simulink model "TargetSpeedThrottle"  (R2021a)
settings: Solver=FixedStepDiscrete  StartTime=0.0  StopTime=10.0  FixedStep=0.01  RelTol=1e-3
undefined symbols (not defined in the file): DiscIntNeverNeededParam, Kp, opMode, target_dec_hold, target_dec_short, target_inc_hold, target_inc_short, throt_max, throt_min, Ts, tsp_max, tsp_min
libraries: simulink x7
settings Model: RequirementInfo={} %GIDa_1a3689c1_601b_4931_a17a_efea0d5071ba  DataDictionary=crs_controllerdic.sldd  EnableAccessToBaseWorkspace=off  Creator=The MathWorks, Inc.  LastModifiedBy=shayashi
settings SolverCC: AlgebraicLoopSolver=TrustRegion
settings DataIOCC: SaveOutput=off  SignalLogging=off  DSMLogging=off  SaveTime=off  ReturnWorkspaceOutputs=off
settings OptimizationCC: DefaultParameterBehavior=Inlined  PassReuseOutputArgsAs=Individual arguments  EfficientTunableParamExpr=on
settings DebuggingCC: ParameterTunabilityLossMsg=error  SFMachineParentedDataDiag=warning  ArithmeticOperatorsInVariantConditions=warning
settings SFSimCC: SimUseLocalCustomCode=off  CustomCodeUndefinedFunction=UseInterfaceOnly
settings RTWCC: SystemTargetFile=ert.tlc  GenCodeOnly=on  TemplateMakefile=ert_default_tmf  GenerateReport=on  RTWUseLocalCustomCode=off  IncludeHyperlinkInReport=on  LaunchReport=on  GenerateTraceInfo=on  GenerateTraceReport=on  GenerateTraceReportSl=on  GenerateTraceReportSf=on  GenerateTraceReportEml=on
settings CodeAppCC: ForceParamTrailComments=on  IgnoreCustomStorageClasses=off  OperatorAnnotations=on  SimulinkDataObjDesc=on  SFDataObjDesc=on  MATLABFcnDesc=on  InsertBlockDesc=on  StateflowObjectComments=on  MATLABSourceComments=on  ReqsInCode=on
settings ERTTargetCC: TargetLangStandard=C99 (ISO)  GenerateSampleERTMain=on  InlinedParameterPlacement=NonHierarchical  ERTCustomFileTemplate=example_file_process.tlc
settings ConfigComp: DVTestSuiteOptimization=Auto  DVDetectOutOfBounds=on

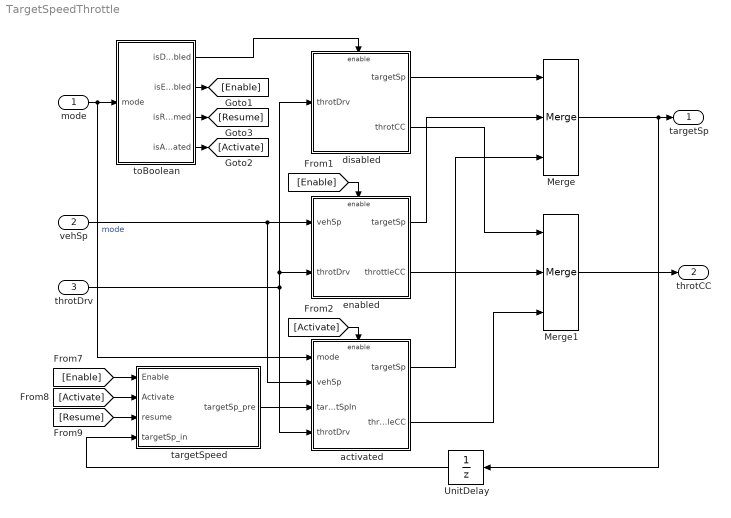
== system TargetSpeedThrottle ==
  mode : Inport  RequirementInfo={} %GIDa_22885af7_b22a_44fa_aa4d_017be81ce3db  OutDataTypeStr=Enum: opMode  PortDimensions=1  SampleTime=[0.01,0]
  vehSp : Inport  RequirementInfo={} %GIDa_f5c97d85_f23b_4cf3_86c5_8760a45faeb2  Port=2  OutDataTypeStr=double  PortDimensions=1  SampleTime=[0.01,0]
  throtDrv : Inport  RequirementInfo={} %GIDa_53068002_6435_432c_bd84_5ec1757fd185  Port=3  OutDataTypeStr=double  PortDimensions=1  SampleTime=[0.01,0]
  Merge : Merge  RequirementInfo={} %GIDa_cdca348c_f4ee_415b_942c_f6cd5980ed22  Inputs=3
  Merge1 : Merge  RequirementInfo={} %GIDa_34b46d63_1e8a_4844_895f_7afabcfedfbe  Inputs=3
  UnitDelay : UnitDelay  RequirementInfo={} %GIDa_36ca9bee_c418_49b5_b025_5c47d96671ca  SampleTime=-1  HasFrameUpgradeWarning=on
      settings: AttributesFormatString=Init = %<InitialCondition>
  activated : Subsystem  RequirementInfo={} %GIDa_d3fc8234_37e6_4215_9250_2cfb9e78a153  TreatAsAtomicUnit=on
  disabled : Subsystem  RequirementInfo={} %GIDa_06140de0_e8d8_402c_b038_77cf0712a248  TreatAsAtomicUnit=on
  enabled : Subsystem  RequirementInfo={} %GIDa_3f53baab_40ad_4365_8baf_4957a2682033  TreatAsAtomicUnit=on
  targetSpeed : Subsystem  RequirementInfo={} %GIDa_cb3d74aa_bbef_46cf_9d83_92915d058f40
  toBoolean : Subsystem  RequirementInfo={} %GIDa_708419c1_1127_4954_9632_16e4105ce24a
  targetSp : Outport  RequirementInfo={} %GIDa_29007791_7843_4644_8d92_505ff71faba5  OutDataTypeStr=double  PortDimensions=1  SampleTime=[0.01,0]  VectorParamsAs1DForOutWhenUnconnected=off
  throtCC : Outport  RequirementInfo={} %GIDa_070a8361_0cd1_420b_a715_f329e916e1ad  Port=2  OutDataTypeStr=double  PortDimensions=1  SampleTime=[0.01,0]  VectorParamsAs1DForOutWhenUnconnected=off
  wires:
  [Activate] -> targetSpeed/2(Activate)
  [Enable] -> targetSpeed/1(Enable)
  targetSpeed/1(targetSp_pre) -> activated/3(targetSpIn)
  mode/1 -> activated/1(mode), toBoolean/1(mode)  "mode"
  [Activate] -> activated/Enable
  [Enable] -> enabled/Enable
  toBoolean/1(isDisabled) -> disabled/Enable
  UnitDelay/1 -> targetSpeed/4(targetSp_in)
  Merge/1 -> UnitDelay/1, targetSp/1
  throtDrv/1 -> activated/4(throtDrv), enabled/2(throtDrv), disabled/1(throtDrv)
  vehSp/1 -> enabled/1(vehSp), activated/2(vehSp)
  toBoolean/2(isEnabled) -> [Enable]
  toBoolean/3(isResumed) -> [Resume]
  toBoolean/4(isActivated) -> [Activate]
  [Resume] -> targetSpeed/3(resume)
  disabled/1(targetSp) -> Merge/1
  enabled/1(targetSp) -> Merge/2
  activated/1(targetSp) -> Merge/3
  activated/2(throttleCC) -> Merge1/3
  enabled/2(throttleCC) -> Merge1/2
  disabled/2(throtCC) -> Merge1/1
  Merge1/1 -> throtCC/1

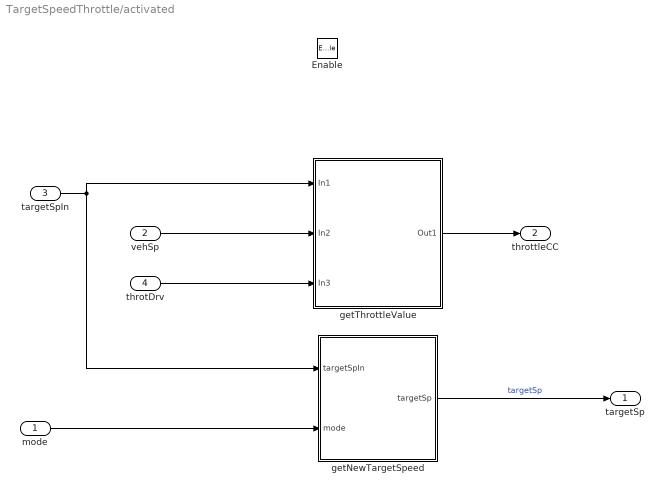
== system TargetSpeedThrottle/activated ==
  mode : Inport  RequirementInfo={} %GIDa_64384464_a4fb_41bc_9e66_5cfe7553856c
  vehSp : Inport  RequirementInfo={} %GIDa_54e68108_b78c_4afe_bc67_449efdb277bd  Port=2
  targetSpIn : Inport  RequirementInfo={} %GIDa_feedb564_4ae2_4bad_9ab3_cf1210728889  Port=3
  throtDrv : Inport  RequirementInfo={} %GIDa_834fa2e2_d354_4482_989f_6165ef52fb64  Port=4
  Enable : EnablePort  RequirementInfo={} %GIDa_bd587e7b_2324_4a3e_a90d_e93b85140e69
  getNewTargetSpeed : Subsystem  RequirementInfo={} %GIDa_cb2db30c_40f4_4c69_83f3_f6a6c8c4dbbc
  getThrottleValue : Subsystem  RequirementInfo={} %GIDa_30fb74e3_5bea_4a48_8902_fa86193af843
  targetSp : Outport  RequirementInfo={} %GIDa_4f1af6e7_9967_48df_a5c8_7598c889d755  VectorParamsAs1DForOutWhenUnconnected=off
  throttleCC : Outport  RequirementInfo={} %GIDa_61cc87ec_8da1_409c_a066_e137f06790c0  Port=2  VectorParamsAs1DForOutWhenUnconnected=off
  wires:
  getThrottleValue/1(Out1) -> throttleCC/1
  throtDrv/1 -> getThrottleValue/3(In3)
  vehSp/1 -> getThrottleValue/2(In2)
  getNewTargetSpeed/1(targetSp) -> targetSp/1  "targetSp"
  mode/1 -> getNewTargetSpeed/2(mode)
  targetSpIn/1 -> getNewTargetSpeed/1(targetSpIn), getThrottleValue/1(In1)

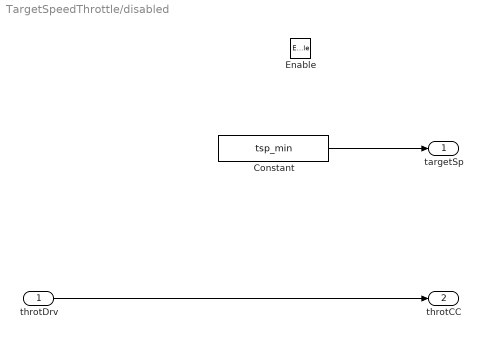
== system TargetSpeedThrottle/disabled ==
  throtDrv : Inport  RequirementInfo={} %GIDa_6cc9cf71_2141_4b22_a535_628638b2431f
  Enable : EnablePort  RequirementInfo={} %GIDa_12e821c3_8a9d_4a2d_ae26_f8ea4cd80d03
  Constant : Constant  RequirementInfo={} %GIDa_549ea7b0_4d18_4b4b_b86d_6f4ed7933c4d  Value=tsp_min  OutDataTypeStr=Inherit: Inherit via back propagation
  targetSp : Outport  RequirementInfo={} %GIDa_cfb9ce1a_28c4_4b9c_a057_b42ee2940ceb  VectorParamsAs1DForOutWhenUnconnected=off
  throtCC : Outport  RequirementInfo={} %GIDa_b0b7c855_10e5_48f0_a23b_03d9ab7ebd64  Port=2  VectorParamsAs1DForOutWhenUnconnected=off
  wires:
  throtDrv/1 -> throtCC/1
  Constant/1 -> targetSp/1

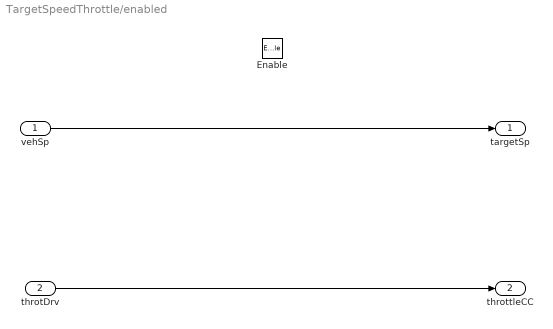
== system TargetSpeedThrottle/enabled ==
  vehSp : Inport  RequirementInfo={} %GIDa_051cacd1_d8f3_45f0_98cd_ed6e0d7dd9aa
  throtDrv : Inport  RequirementInfo={} %GIDa_4482214a_b082_4025_affc_42904b284b10  Port=2
  Enable : EnablePort  RequirementInfo={} %GIDa_6682126c_96c9_4657_ae5d_14402d8b3ec1
  targetSp : Outport  RequirementInfo={} %GIDa_6209277a_e70a_46cf_9111_d4ad6ceba119  VectorParamsAs1DForOutWhenUnconnected=off
  throttleCC : Outport  RequirementInfo={} %GIDa_5cd745c9_300b_4598_b460_5fe843c280e4  Port=2  VectorParamsAs1DForOutWhenUnconnected=off
  wires:
  throtDrv/1 -> throttleCC/1
  vehSp/1 -> targetSp/1

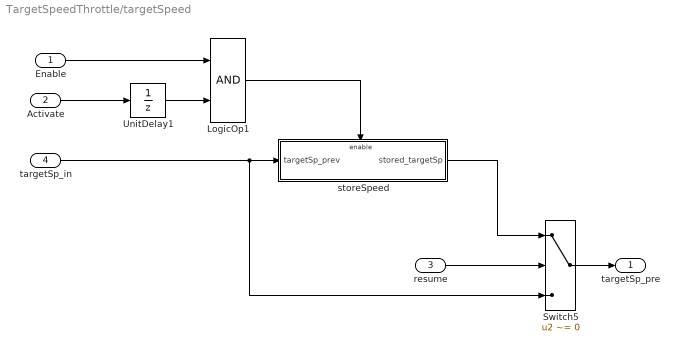
== system TargetSpeedThrottle/targetSpeed ==
  Enable : Inport  RequirementInfo={} %GIDa_fce2bafd_f2de_42bd_8112_e657c8fe1477
  Activate : Inport  RequirementInfo={} %GIDa_8a860952_06c5_4d89_b310_dabeeaa78df6  Port=2
  resume : Inport  RequirementInfo={} %GIDa_d24781cb_7428_4781_b55e_e26f6e81c793  Port=3
  targetSp_in : Inport  RequirementInfo={} %GIDa_97c5bf71_ad17_419d_a89a_c68daaf71e8b  Port=4
  LogicOp1 : Logic  RequirementInfo={} %GIDa_9c82f171_f4c6_4d19_9b0e_13b686137bc8  AllPortsSameDT=off  OutDataTypeStr=boolean
  Switch5 : Switch  RequirementInfo={} %GIDa_9efa5802_f260_41d2_9ca5_821b46ab96a6  Criteria=u2 ~= 0
  UnitDelay1 : UnitDelay  RequirementInfo={} %GIDa_adabed4e_2068_480c_8557_03c012030ff1  InitialCondition=false  SampleTime=-1  HasFrameUpgradeWarning=on
      settings: AttributesFormatString=Init = %<InitialCondition>
  storeSpeed : Subsystem  RequirementInfo={} %GIDa_21626e59_d900_4aed_83eb_aaced630845b  TreatAsAtomicUnit=on
  targetSp_pre : Outport  RequirementInfo={} %GIDa_7bb45878_dbc3_4fb7_871d_d80e6eee27c9  VectorParamsAs1DForOutWhenUnconnected=off
  wires:
  Switch5/1 -> targetSp_pre/1
  targetSp_in/1 -> storeSpeed/1(targetSp_prev), Switch5/3
  resume/1 -> Switch5/2
  Enable/1 -> LogicOp1/1
  LogicOp1/1 -> storeSpeed/Enable
  UnitDelay1/1 -> LogicOp1/2
  Activate/1 -> UnitDelay1/1
  storeSpeed/1(stored_targetSp) -> Switch5/1

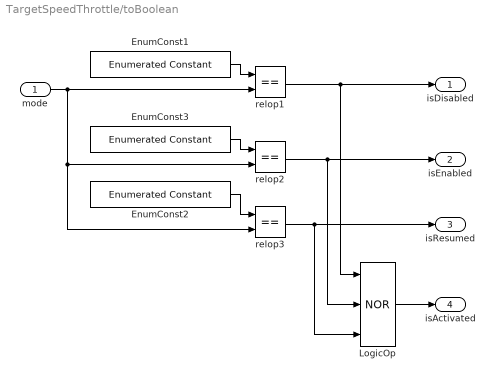
== system TargetSpeedThrottle/toBoolean ==
  mode : Inport  RequirementInfo={} %GIDa_e7e444c0_3529_4ed5_81ce_f617e2024f02
  EnumConst1 : simulink/Sources/Enumerated Constant  RequirementInfo={} %GIDa_27a9e84b_6b36_4c12_aa93_aca0a05eed93  OutDataTypeStr=Enum: opMode  Value=opMode.Disable  SampleTime=inf
  EnumConst2 : simulink/Sources/Enumerated Constant  RequirementInfo={} %GIDa_d37b8a40_9443_4f54_8bef_716a0ad75842  OutDataTypeStr=Enum: opMode  Value=opMode.Resume  SampleTime=inf
  EnumConst3 : simulink/Sources/Enumerated Constant  RequirementInfo={} %GIDa_e76c0d8e_43de_4bf9_b183_6cfd99518f27  OutDataTypeStr=Enum: opMode  Value=opMode.Enable  SampleTime=inf
  LogicOp : Logic  RequirementInfo={} %GIDa_c0c1558f_e301_4739_9f83_d240660de869  Operator=NOR  Inputs=3  AllPortsSameDT=off  OutDataTypeStr=boolean
  relop1 : RelationalOperator  RequirementInfo={} %GIDa_8114262e_aab4_4130_b326_8c0e06239675  Operator===  OutDataTypeStr=boolean  RndMeth=Nearest
  relop2 : RelationalOperator  RequirementInfo={} %GIDa_f220986f_8ed3_4e7b_a738_7af982ee01f8  Operator===  OutDataTypeStr=boolean  RndMeth=Nearest
  relop3 : RelationalOperator  RequirementInfo={} %GIDa_2bb1450f_1cf8_4106_805d_3854b6e18c7a  Operator===  OutDataTypeStr=boolean  RndMeth=Nearest
  isDisabled : Outport  RequirementInfo={} %GIDa_0a060732_89ab_4bb9_8b58_ea59ba79c186  VectorParamsAs1DForOutWhenUnconnected=off
  isEnabled : Outport  RequirementInfo={} %GIDa_daac9f50_969b_4fdf_9786_3d46f846d53d  Port=2  VectorParamsAs1DForOutWhenUnconnected=off
  isResumed : Outport  RequirementInfo={} %GIDa_93357058_38d0_4ce0_963d_ef84644f8231  Port=3  VectorParamsAs1DForOutWhenUnconnected=off
  isActivated : Outport  RequirementInfo={} %GIDa_74b726ca_5975_4bda_b81c_40dfcc9ca42e  Port=4  VectorParamsAs1DForOutWhenUnconnected=off
  wires:
  mode/1 -> relop1/2, relop3/2, relop2/2
  EnumConst1/1 -> relop1/1
  relop1/1 -> LogicOp/1, isDisabled/1
  EnumConst3/1 -> relop2/1
  relop2/1 -> LogicOp/2, isEnabled/1
  LogicOp/1 -> isActivated/1
  EnumConst2/1 -> relop3/1
  relop3/1 -> LogicOp/3, isResumed/1

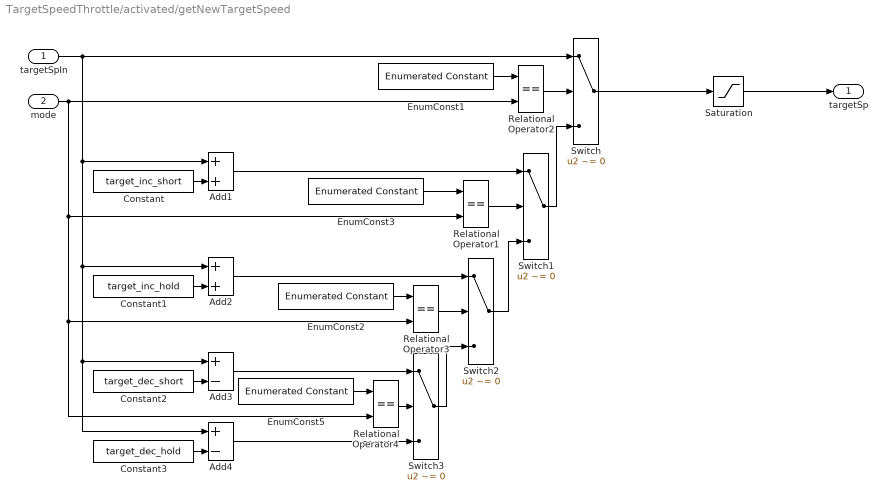
== system TargetSpeedThrottle/activated/getNewTargetSpeed ==
  targetSpIn : Inport  RequirementInfo={} %GIDa_dd8112e1_43c3_4a47_90be_f2c55a92c62c
  mode : Inport  RequirementInfo={} %GIDa_b2b77f36_22c4_4b18_ac87_18cb3421a625  Port=2
  Add1 : Sum  RequirementInfo={} %GIDa_ab25794c_4e33_4e3f_847d_a22081c840de
  Add2 : Sum  RequirementInfo={} %GIDa_5ea28e83_3a91_4ee0_8d0c_1ce0d3410099
  Add3 : Sum  RequirementInfo={} %GIDa_d3818476_c517_41f9_9138_95667138fdaf  Inputs=+-
  Add4 : Sum  RequirementInfo={} %GIDa_cac1df21_bf31_404f_a3d2_04b0d0e259f5  Inputs=+-
  Constant : Constant  RequirementInfo={} %GIDa_685e717d_0e07_4cad_af9d_a79c0745fc95  Value=target_inc_short  OutDataTypeStr=Inherit: Inherit via back propagation
  Constant1 : Constant  RequirementInfo={} %GIDa_3382b574_f6a4_429e_846e_9c5ac42ab0c9  Value=target_inc_hold  OutDataTypeStr=Inherit: Inherit via back propagation
  Constant2 : Constant  RequirementInfo={} %GIDa_0a83c9ff_2402_4538_b8c0_89582db4bec9  Value=target_dec_short  OutDataTypeStr=Inherit: Inherit via back propagation
  Constant3 : Constant  RequirementInfo={} %GIDa_375ab84b_74bf_4a19_bb7b_71dc43b7dd75  Value=target_dec_hold  OutDataTypeStr=Inherit: Inherit via back propagation
  EnumConst1 : simulink/Sources/Enumerated Constant  RequirementInfo={} %GIDa_e916a5d7_1f9c_403a_9fb5_c68eafe47a3d  OutDataTypeStr=Enum: opMode  Value=opMode.Activate  SampleTime=inf
  EnumConst2 : simulink/Sources/Enumerated Constant  RequirementInfo={} %GIDa_3c7e951b_786e_4a67_9f5a_7a15f406886c  OutDataTypeStr=Enum: opMode  Value=opMode.IncrementHold  SampleTime=inf
  EnumConst3 : simulink/Sources/Enumerated Constant  RequirementInfo={} %GIDa_18669ea9_4413_413e_8bff_adabad1b4fbd  OutDataTypeStr=Enum: opMode  Value=opMode.Increment  SampleTime=inf
  EnumConst5 : simulink/Sources/Enumerated Constant  RequirementInfo={} %GIDa_912f467c_312f_4c35_abfa_b674e7bf14ca  OutDataTypeStr=Enum: opMode  Value=opMode.Decrement  SampleTime=inf
  Relational Operator1 : RelationalOperator  RequirementInfo={} %GIDa_2bf2086d_3dd7_43ee_85b8_aed8a3106e89  Operator===  OutDataTypeStr=boolean  RndMeth=Nearest
  Relational Operator2 : RelationalOperator  RequirementInfo={} %GIDa_1501cc1d_d17d_4708_8783_1677c4f8962d  Operator===  OutDataTypeStr=boolean  RndMeth=Nearest
  Relational Operator3 : RelationalOperator  RequirementInfo={} %GIDa_ed0be5fa_63ee_43b0_8875_05b5aa8618a9  Operator===  OutDataTypeStr=boolean  RndMeth=Nearest
  Relational Operator4 : RelationalOperator  RequirementInfo={} %GIDa_0c957258_9518_4932_94c2_55668310b467  Operator===  OutDataTypeStr=boolean  RndMeth=Nearest
  Saturation : Saturate  RequirementInfo={} %GIDa_638d5f71_5582_42aa_a38b_771c9465ce6d  UpperLimit=tsp_max  LowerLimit=tsp_min
      settings: AttributesFormatString=|
      | H:%<UpperLimit>
      | L:%<LowerLimit>
  Switch : Switch  RequirementInfo={} %GIDa_9f9dca14_7851_4d61_9187_7989930f11a0  Criteria=u2 ~= 0
  Switch1 : Switch  RequirementInfo={} %GIDa_8092d072_0606_4649_9f7e_ec276ef4a20b  Criteria=u2 ~= 0
  Switch2 : Switch  RequirementInfo={} %GIDa_2de9aa0a_ebdf_4c3a_9d62_e41fcd8865a2  Criteria=u2 ~= 0
  Switch3 : Switch  RequirementInfo={} %GIDa_55554a55_8461_4935_922b_f6be856ad7f1  Criteria=u2 ~= 0
  targetSp : Outport  RequirementInfo={} %GIDa_bf662dca_49c4_4c09_b940_056f915f0760  VectorParamsAs1DForOutWhenUnconnected=off
  wires:
  Saturation/1 -> targetSp/1
  Relational Operator2/1 -> Switch/2
  Switch/1 -> Saturation/1
  Relational Operator1/1 -> Switch1/2
  Switch1/1 -> Switch/3
  Switch2/1 -> Switch1/3
  Constant/1 -> Add1/2
  Relational Operator3/1 -> Switch2/2
  Add1/1 -> Switch1/1
  Add2/1 -> Switch2/1
  Constant1/1 -> Add2/2
  Add3/1 -> Switch3/1
  Relational Operator4/1 -> Switch3/2
  EnumConst5/1 -> Relational Operator4/1
  Constant2/1 -> Add3/2
  Constant3/1 -> Add4/2
  EnumConst3/1 -> Relational Operator1/1
  EnumConst1/1 -> Relational Operator2/1
  mode/1 -> Relational Operator2/2, Relational Operator1/2, Relational Operator3/2, Relational Operator4/2
  EnumConst2/1 -> Relational Operator3/1
  Add4/1 -> Switch3/3
  Switch3/1 -> Switch2/3
  targetSpIn/1 -> Add2/1, Add3/1, Add4/1, Add1/1, Switch/1

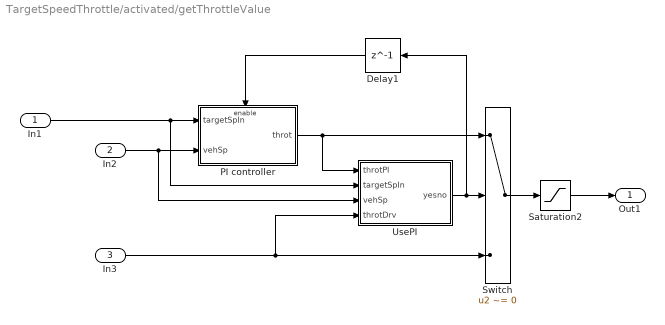
== system TargetSpeedThrottle/activated/getThrottleValue ==
  In1 : Inport  RequirementInfo={} %GIDa_061496d3_fee6_49dd_b810_9e181e5a4467
  In2 : Inport  RequirementInfo={} %GIDa_0ea5875c_2ec6_418e_bb1e_c4c70a87c7e8  Port=2
  In3 : Inport  RequirementInfo={} %GIDa_62b27e0c_7f2b_474c_98d5_6e7de758dbd9  Port=3
  Delay1 : Delay  RequirementInfo={} %GIDa_bbcfe40d_0a59_4ed0_ab59_8d6beb5a6bc3  DelayLength=1  InitialCondition=0
      settings: AttributesFormatString=Init = %<InitialCondition>
  PI controller : Subsystem  RequirementInfo={} %GIDa_858910af_ba13_4cbf_b633_ef2ac9ec12a4  TreatAsAtomicUnit=on
  Saturation2 : Saturate  RequirementInfo={} %GIDa_a8362d82_50ad_42bf_91cd_8463692ac67c  UpperLimit=throt_max  LowerLimit=throt_min
      settings: AttributesFormatString=|
      | H:%<UpperLimit>
      | L:%<LowerLimit>
  Switch : Switch  RequirementInfo={} %GIDa_0f358fe5_a21a_47a6_92db_538a5f4972b3  Criteria=u2 ~= 0
  UsePI : Subsystem  RequirementInfo={} %GIDa_325fb434_7baf_41b2_8f9d_97e5a51370b7
  Out1 : Outport  RequirementInfo={} %GIDa_73cf9ec6_f528_4bf7_ae7f_c880a3ad5903  VectorParamsAs1DForOutWhenUnconnected=off
  wires:
  In1/1 -> PI controller/1(targetSpIn), UsePI/2(targetSpIn)
  Switch/1 -> Saturation2/1
  PI controller/1(throt) -> Switch/1, UsePI/1(throtPI)
  Saturation2/1 -> Out1/1
  In2/1 -> PI controller/2(vehSp), UsePI/3(vehSp)
  UsePI/1(yesno) -> Switch/2, Delay1/1
  Delay1/1 -> PI controller/Enable
  In3/1 -> Switch/3, UsePI/4(throtDrv)

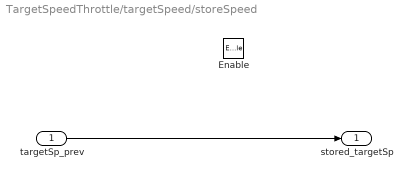
== system TargetSpeedThrottle/targetSpeed/storeSpeed ==
  targetSp_prev : Inport  RequirementInfo={} %GIDa_50ee833c_e8f7_4fbc_85c4_0ec4dcaaeffd
  Enable : EnablePort  RequirementInfo={} %GIDa_4d20878e_22e5_41e6_9d85_98d24833a217
  stored_targetSp : Outport  RequirementInfo={} %GIDa_a13c37f3_e319_4efa_99c2_10cac7bbdea5  VectorParamsAs1DForOutWhenUnconnected=off
  wires:
  targetSp_prev/1 -> stored_targetSp/1

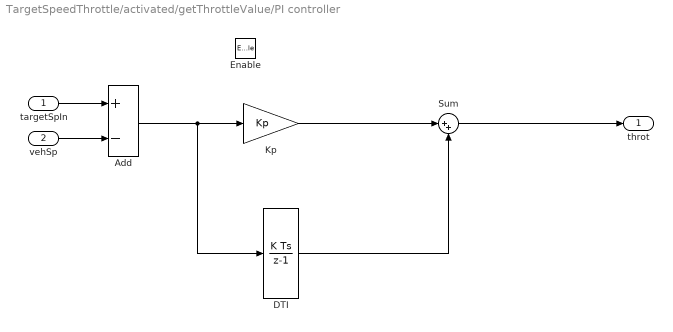
== system TargetSpeedThrottle/activated/getThrottleValue/PI controller ==
  targetSpIn : Inport  RequirementInfo={} %GIDa_93a3cc3d_44a3_44c5_9669_fde66396f4b2
  vehSp : Inport  RequirementInfo={} %GIDa_b8b25f09_7eb2_4e20_8f87_ca43fffb4cc3  Port=2
  Enable : EnablePort  RequirementInfo={} %GIDa_4ccb8e77_795e_4c72_951f_5a32b6f81975  StatesWhenEnabling=reset
  Add : Sum  RequirementInfo={} %GIDa_b19ed4bc_0bfb_4e5d_b402_c1475401def1  Inputs=+-
  "DTI " : DiscreteIntegrator  RequirementInfo={} %GIDa_7694b4f6_1105_4f90_8b40_037bb89038a6  gainval=Ki  SampleTime=Ts  ICPrevOutput=DiscIntNeverNeededParam  ICPrevScaledInput=DiscIntNeverNeededParam
  Kp : Gain  RequirementInfo={} %GIDa_537ac4b2_5d63_4200_9528_2e488c8e1c16  Gain=Kp
  Sum : Sum  RequirementInfo={} %GIDa_f46968c2_b58a_4f4c_8eb9_11e4e56906ac  Inputs=|++
  throt : Outport  RequirementInfo={} %GIDa_777969f7_9e90_4ddc_95cd_a4e630dd8c6a  OutputWhenDisabled=reset  InitialOutput=0  VectorParamsAs1DForOutWhenUnconnected=off
  wires:
  vehSp/1 -> Add/2
  targetSpIn/1 -> Add/1
  Add/1 -> Kp/1, "DTI "/1
  Sum/1 -> throt/1
  "DTI "/1 -> Sum/2
  Kp/1 -> Sum/1

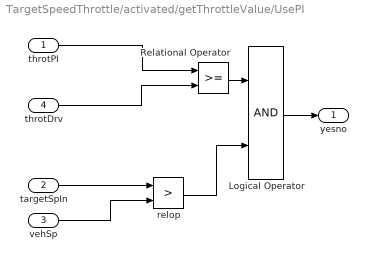
== system TargetSpeedThrottle/activated/getThrottleValue/UsePI ==
  throtPI : Inport  RequirementInfo={} %GIDa_24ab5ede_d8f1_4bee_8be2_95b608e3fd7e
  targetSpIn : Inport  RequirementInfo={} %GIDa_e08332c5_06cc_4f3c_9f86_00235894ed60  Port=2
  vehSp : Inport  RequirementInfo={} %GIDa_ba55cb28_ab2e_457b_9793_377830b25f08  Port=3
  throtDrv : Inport  RequirementInfo={} %GIDa_caf261da_81df_4664_ba68_c1d339104b09  Port=4
  Logical Operator : Logic  RequirementInfo={} %GIDa_b44fe4db_bbfc_490d_b671_58da8530985a  AllPortsSameDT=off  OutDataTypeStr=boolean
  Relational Operator : RelationalOperator  RequirementInfo={} %GIDa_c9af3f80_509d_4b2b_bb74_49874574d420  OutDataTypeStr=boolean  RndMeth=Nearest
  relop : RelationalOperator  RequirementInfo={} %GIDa_fef9c1e3_cb16_46b7_ba92_752ba66c74f6  Operator=>  OutDataTypeStr=boolean  RndMeth=Nearest
  yesno : Outport  RequirementInfo={} %GIDa_d9e96a20_2915_4294_845e_2559c8521615  VectorParamsAs1DForOutWhenUnconnected=off
  wires:
  throtPI/1 -> Relational Operator/1
  vehSp/1 -> relop/2
  targetSpIn/1 -> relop/1
  throtDrv/1 -> Relational Operator/2
  Logical Operator/1 -> yesno/1
  relop/1 -> Logical Operator/2
  Relational Operator/1 -> Logical Operator/1
